simulink library "powerlib_modelsV2"  (Simulink 6.0)
settings: Solver=ode45  SolverMode=SingleTasking  StartTime=0.0  StopTime=10.0  RelTol=1e-3
values from neighbouring files (symbols this model uses):
  Ts = get(handles.edit1,'string')    [powergui.m]
undefined symbols (not defined in the file or in its folder): A, Ac, B, Bc, C, Cc, Cs, Current, damp, Dc, Dd, DiscIntNeverNeededParam, dref, dwo, exc, F, fb, gate, GH, GHd, GI, GId, GL, GLd, H, HT, hyd, ib, ib2, io, isfinite, j, K, Kd, Kg, L, Lad, Laq, lim, LIM, Ll, Llfd, Llkd, Llkq1, Llkq2, Llr, Lls, LowerFlux, N, N2, Nb, Nb2, nb_arm, p, Par_HarmoA_pu, Par_HarmoB_pu, Par_Timing_Harmo, Par_Timing_Variation, Par_Vps, Pb ... (+57)
libraries: powerlib_extras x14
(part 5 of 11)

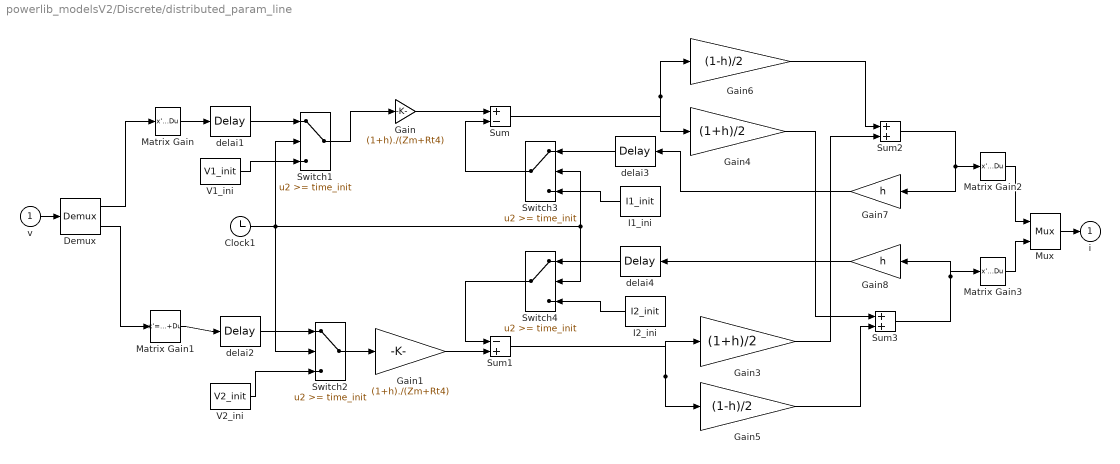
== system powerlib_modelsV2/Discrete/distributed_param_line ==
  v : Inport  Port=1  LatchInput=off
  Clock1 : Clock
      settings: Decimation=10
  Demux : Demux  Outputs=[nphase,nphase]
  Gain : Gain  Gain=(1+h)./(Zm+Rt4)  SaturateOnIntegerOverflow=on
  Gain1 : Gain  Gain=(1+h)./(Zm+Rt4)  SaturateOnIntegerOverflow=on
  Gain3 : Gain  Gain=(1+h)/2  SaturateOnIntegerOverflow=on
  Gain4 : Gain  Gain=(1+h)/2  SaturateOnIntegerOverflow=on
  Gain5 : Gain  Gain=(1-h)/2  SaturateOnIntegerOverflow=on
  Gain6 : Gain  Gain=(1-h)/2  SaturateOnIntegerOverflow=on
  Gain7 : Gain  Orientation=left  Gain=h  SaturateOnIntegerOverflow=on
  Gain8 : Gain  Orientation=left  Gain=h  SaturateOnIntegerOverflow=on
  I1_ini : FromWorkspace  Orientation=left  VariableName=I1_init  SampleTime=0
  I2_ini : FromWorkspace  Orientation=left  VariableName=I2_init  SampleTime=0
  Matrix Gain : StateSpace  A=[]  B=[]  C=[]  D=K  mask(Matrix Gain){@1=Ti'}
      mask prompts: @1 "Gain matrix:"
      mask help: Matrix Gain.
      mask init:
      | K = @1;
      mask Help: Multiplies input vector by entered matrix to produce output vector (y=Au).
      mask Display: disp('K')
  Matrix Gain1 : StateSpace  A=[]  B=[]  C=[]  D=K  mask(Matrix Gain){@1=Ti'}
      mask prompts: @1 "Gain matrix:"
      mask help: Matrix Gain.
      mask init:
      | K = @1;
      mask Help: Multiplies input vector by entered matrix to produce output vector (y=Au).
      mask Display: disp('K')
  Matrix Gain2 : StateSpace  A=[]  B=[]  C=[]  D=K  mask(Matrix Gain){@1=Ti}
      mask prompts: @1 "Gain matrix:"
      mask help: Matrix Gain.
      mask init:
      | K = @1;
      mask Help: Multiplies input vector by entered matrix to produce output vector (y=Au).
      mask Display: disp('K')
  Matrix Gain3 : StateSpace  A=[]  B=[]  C=[]  D=K  mask(Matrix Gain){@1=Ti}
      mask prompts: @1 "Gain matrix:"
      mask help: Matrix Gain.
      mask init:
      | K = @1;
      mask Help: Multiplies input vector by entered matrix to produce output vector (y=Au).
      mask Display: disp('K')
  Mux : Mux  Inputs=[nphase,nphase]
  Sum : Sum  Inputs=+-  SaturateOnIntegerOverflow=on  InputSameDT=on
  Sum1 : Sum  Inputs=-+  SaturateOnIntegerOverflow=on  InputSameDT=on
  Sum2 : Sum  SaturateOnIntegerOverflow=on  InputSameDT=on
  Sum3 : Sum  SaturateOnIntegerOverflow=on  InputSameDT=on
  Switch1 : Switch  Threshold=time_init  InputSameDT=on
  Switch2 : Switch  Threshold=time_init  InputSameDT=on
  Switch3 : Switch  Orientation=left  Threshold=time_init  InputSameDT=on
  Switch4 : Switch  Orientation=left  Threshold=time_init  InputSameDT=on
  V1_ini : FromWorkspace  VariableName=V1_init  SampleTime=0
  V2_ini : FromWorkspace  VariableName=V2_init  SampleTime=0
  delai1 : TransportDelay  DelayTime=to
  delai2 : TransportDelay  DelayTime=to
  delai3 : TransportDelay  Orientation=left  DelayTime=to
  delai4 : TransportDelay  Orientation=left  DelayTime=to
  i : Outport  InitialOutput=0
  wires:
  I2_ini/1 -> Switch4/3
  I1_ini/1 -> Switch3/3
  Clock1/1 -> Switch1/2, Switch2/2, Switch3/2, Switch4/2
  delai4/1 -> Switch4/1
  Switch4/1 -> Sum1/1
  Switch3/1 -> Sum/2
  delai3/1 -> Switch3/1
  Sum1/1 -> Gain5/1, Gain3/1
  Sum/1 -> Gain6/1, Gain4/1
  V2_ini/1 -> Switch2/3
  delai2/1 -> Switch2/1
  Switch1/1 -> Gain/1
  Switch2/1 -> Gain1/1
  V1_ini/1 -> Switch1/3
  delai1/1 -> Switch1/1
  Gain8/1 -> delai4/1
  Sum2/1 -> Matrix Gain2/1, Gain7/1
  Gain7/1 -> delai3/1
  Sum3/1 -> Matrix Gain3/1, Gain8/1
  Mux/1 -> i/1
  v/1 -> Demux/1
  Gain1/1 -> Sum1/2
  Gain/1 -> Sum/1
  Gain5/1 -> Sum3/2
  Gain6/1 -> Sum2/1
  Gain3/1 -> Sum2/2
  Gain4/1 -> Sum3/1
  Matrix Gain/1 -> delai1/1
  Demux/1 -> Matrix Gain/1
  Matrix Gain1/1 -> delai2/1
  Demux/2 -> Matrix Gain1/1
  Matrix Gain3/1 -> Mux/2
  Matrix Gain2/1 -> Mux/1

== system powerlib_modelsV2/Discrete/hysteresis_transformer ==
  v : Inport  Port=1  LatchInput=off
  Hysteresis ( always in SI ) : Subsystem
  fluxinit : DiscreteIntegrator  IntegratorMethod=Integration: Backward Euler  InitialCondition=fluxinit  SampleTime=Ts  SaturateOnIntegerOverflow=on  ICPrevOutput=DiscIntNeverNeededParam  ICPrevScaledInput=DiscIntNeverNeededParam
  i : Outport  InitialOutput=0
  f : Outport  Port=2  InitialOutput=0
  wires:
  v/1 -> fluxinit/1
  fluxinit/1 -> f/1, Hysteresis ( always in SI )/1(In1)  "flux displayed by Multimeter block"
  Hysteresis ( always in SI )/1(Out1) -> i/1

== system powerlib_modelsV2/Discrete/ideal_switch ==
  v : Inport  Port=1  LatchInput=off
  g : Inport  Port=2  LatchInput=off
  0 1 : Constant  Value=0
  Constant : Constant  Value=zeros(Nsw,1)
  Data Type Conversion1 : DataTypeConversion  SaturateOnIntegerOverflow=on  RndMeth=Zero
  Gain : Gain  Gain=1./Rsw  SaturateOnIntegerOverflow=on
  Mux : Mux  Inputs=2
  Switch : Switch  Threshold=0.5  InputSameDT=on
  i : Outport  InitialOutput=0
  Status : Outport  Port=2  InitialOutput=0
  m : Outport  Port=3  InitialOutput=0
  wires:
  v/1 -> Mux/2, Gain/1  "Vak"
  Mux/1 -> m/1  "measurement signals"
  g/1 -> Switch/2, Data Type Conversion1/1
  Constant/1 -> i/1
  Switch/1 -> Mux/1
  Gain/1 -> Switch/1  "Iak"
  0 1/1 -> Switch/3
  Data Type Conversion1/1 -> Status/1

== system powerlib_modelsV2/Discrete/saturable_transformer ==
  v : Inport  Port=1  LatchInput=off
  Discrete-Time Integrator : DiscreteIntegrator  IntegratorMethod=Integration: Trapezoidal  InitialCondition=fluxinit  SampleTime=Ts  SaturateOnIntegerOverflow=on  ICPrevOutput=DiscIntNeverNeededParam  ICPrevScaledInput=DiscIntNeverNeededParam
  Look-Up Table : Lookup  DialogController=Simulink.DDGSource  InputValues=phisat  OutputValues=isat  SaturateOnIntegerOverflow=on
  i : Outport  InitialOutput=0
  f : Outport  Port=2  InitialOutput=0
  wires:
  v/1 -> Discrete-Time Integrator/1
  Discrete-Time Integrator/1 -> Look-Up Table/1, f/1
  Look-Up Table/1 -> i/1

== system powerlib_modelsV2/Discrete/simplified_sync_mach ==
  v : Inport  Port=1  LatchInput=off
  pm : Inport  Port=2  LatchInput=off
  e : Inport  Port=3  LatchInput=off
  1\p : Gain  Gain=1/p  SaturateOnIntegerOverflow=on
  Selector : Selector  Elements=sel  InputPortWidth=3
  Subsystem : Subsystem
  Vt : Subsystem
  Z : Subsystem
      mask Display: disp('Z')
  gen : Subsystem
      mask Display: disp('gen')
  ib : Gain  Gain=ib  SaturateOnIntegerOverflow=on
  mechanics : Subsystem
      mask Display: disp('mec')
  wattmeter : Subsystem  Orientation=left
      mask Display: disp('wattmeter')
  i : Outport  InitialOutput=0
  * : Outport  Port=2  InitialOutput=0
  wires:
  Subsystem/1(*) -> */1
  Vt/2(Vabc) -> Subsystem/2(v), Z/2(v)
  Vt/1(Vn) -> gen/3(Vn)
  gen/1(e) -> wattmeter/2(v), Z/1(e), Subsystem/3(e)  "e"
  Z/1(i) -> wattmeter/1(i), Subsystem/1(i), ib/1
  mechanics/2(wm) -> Subsystem/5(wm)
  1\p/1 -> Subsystem/4(theta)
  v/1 -> Vt/1(V)
  mechanics/1(theta_e) -> gen/1(theta), 1\p/1
  e/1 -> gen/2(E)
  pm/1 -> mechanics/1(Pm)
  wattmeter/1(Pe) -> Subsystem/6(Pe), mechanics/2(Pe)
  ib/1 -> Selector/1
  Selector/1 -> i/1

== system powerlib_modelsV2/Discrete/surge_arrester ==
  v : Inport  Port=1  LatchInput=off
  Abs : Abs  SaturateOnIntegerOverflow=on
  Product : Product  SaturateOnIntegerOverflow=on  InputSameDT=on
  Sign : Signum  Orientation=down
  Switch1 : Switch  Threshold=ic1  InputSameDT=on
  Switch2 : Switch  Threshold=ic2  InputSameDT=on
  Unit Delay1 : UnitDelay  SampleTime=Ts
  segment1 : Fcn  Expr=p1*(u/uref)^a1
  segment2 : Fcn  Expr=p2*(u/uref)^a2
  segment3 : Fcn  Expr=p3*(u/uref)^a3
  i : Outport  InitialOutput=0
  wires:
  segment3/1 -> Switch2/1
  Switch1/1 -> Switch2/3, Switch2/2
  Switch2/1 -> Product/1
  segment2/1 -> Switch1/1
  segment1/1 -> Switch1/2, Switch1/3
  Abs/1 -> segment3/1, segment2/1, segment1/1
  Sign/1 -> Product/2
  v/1 -> Abs/1, Sign/1
  Product/1 -> Unit Delay1/1
  Unit Delay1/1 -> i/1

== system powerlib_modelsV2/Discrete/synchronous_machine ==
  v : Inport  Port=1  LatchInput=off
  pm : Inport  Port=2  LatchInput=off
  vf : Inport  Port=3  LatchInput=off
  Delta angle : Subsystem
  Discrete-Time Integrator1 : DiscreteIntegrator  InitialCondition=tho  SampleTime=Ts  SaturateOnIntegerOverflow=on  ICPrevOutput=DiscIntNeverNeededParam  ICPrevScaledInput=DiscIntNeverNeededParam
  Fcn : Fcn  Expr=rem(u,2*pi)
  Mux1 : Mux  Inputs=[ 3 8 2 4 1 1 1 1 1]
  PQ : Subsystem
  Subsystem : Subsystem
  Unit Delay1 : UnitDelay  Orientation=left  X0=phiqo  SampleTime=Ts
  Unit Delay2 : UnitDelay  Orientation=left  X0=phiqo  SampleTime=Ts
  abc2qd : Subsystem
      mask Display: disp('abc/\nqd')
  currents and mutual fluxes : Subsystem
      mask Display: disp('currents\nand\nmutual\nfluxes')
  ia,ib : Selector  Elements=1:2  InputPortWidth=3
  mec : Subsystem
      mask Display: disp('mec')
  output formatting : Gain  Gain=[ib2*ones(1,5),N2,ib2,ib2,ib2,phib,phib,Vb2,Vb2,1,Nb,Pb,1,1,1,1,1,1]
  phid : Subsystem
      mask Display: disp('phid')
  phifd : Subsystem
      mask Display: disp('phifd')
  phikd : Subsystem
      mask Display: disp('phikd')
  phikq1 : Subsystem
      mask Display: disp('phikq1')
  phikq2 : Subsystem
      mask Display: disp('phikq2')
  phiq : Subsystem
      mask Display: disp('phiq')
  qd2abc : Subsystem
      mask Display: disp('qd/\nabc')
  theta : Gain  Gain=180/pi  SaturateOnIntegerOverflow=on
  vkd : Ground
  vkq2 : Ground
  web1 : Gain  Gain=web_psb  SaturateOnIntegerOverflow=on
  i : Outport  InitialOutput=0
  m : Outport  Port=2  InitialOutput=0
  wires:
  Subsystem/2(Vfd) -> phifd/1(vfd)
  Subsystem/1(Vkq1) -> phikq1/2(vkq1)
  phikq2/1(phikq2) -> currents and mutual fluxes/2(phikq2)
  phikq1/1(phikq1) -> currents and mutual fluxes/5(phikq1)
  phifd/1(phifd) -> currents and mutual fluxes/4(phifd)
  phikd/1(phikd) -> currents and mutual fluxes/6(phikd)
  v/1 -> abc2qd/1(v)
  currents and mutual fluxes/4(phimd) -> Unit Delay2/1
  abc2qd/3(vd) -> phid/3(vd), PQ/2(Vd), Delta angle/2(Vd)
  phid/1(phid) -> mec/2(phid), phiq/3(phid), currents and mutual fluxes/3(phid)
  output formatting/1 -> m/1
  ia,ib/1 -> i/1
  Mux1/1 -> output formatting/1
  currents and mutual fluxes/3(iq,id) -> qd2abc/2(iq,id), mec/1("iq,id "), PQ/3(Iq)  "iq,id"
  abc2qd/1(cos,sin) -> qd2abc/1(sin,cos)  "sin,cos"
  abc2qd/4(vq,vd) -> Mux1/3  "vq,vd"
  qd2abc/2(is(pu)) -> Mux1/1  "is(3)"
  mec/1(misc) -> Mux1/4  "d_theta,n,Pe,dw"
  currents and mutual fluxes/1(phimq) -> Unit Delay1/1
  qd2abc/1(is(A)) -> ia,ib/1  "iabc"
  phiq/1(phiq) -> currents and mutual fluxes/1(phiq), mec/3(phiq), phid/2(phiq)
  vkd/1 -> phikd/2(vkd)
  pm/1 -> mec/4(Pm)
  abc2qd/2(vq) -> phiq/1(vq), PQ/1(Vq), Delta angle/1(Vq)
  vkq2/1 -> phikq2/1(vkq2)
  currents and mutual fluxes/2("iq,id,ifd, ikq1,ikq2,ikd, phimq,phimd") -> Mux1/2  "iq,id,ifd,ikq1,ikq2,ikd,phimq,phimd"
  vf/1 -> Subsystem/1(Vf)
  mec/2(thetae) -> abc2qd/2(theta)
  mec/3(we) -> phid/1(w), phiq/2(w), web1/1
  Fcn/1 -> theta/1
  Discrete-Time Integrator1/1 -> Fcn/1
  web1/1 -> Discrete-Time Integrator1/1
  theta/1 -> Mux1/5  "theta"
  Unit Delay1/1 -> phikq1/1(phimq), phikq2/2(phimq), phiq/4(phimq)
  Unit Delay2/1 -> phifd/2(phimd), phikd/1(phimd), phid/4(phimd)
  mec/4("Te ") -> Mux1/6  "Te"
  Delta angle/1(delta) -> Mux1/7
  PQ/1(Peo) -> Mux1/8
  PQ/2(Qeo) -> Mux1/9

== system powerlib_modelsV2/Discrete/thyristor (logical) ==
  note: Current prediction
  v : Inport  Port=1  LatchInput=off
  g : Inport  Port=2  LatchInput=off
  " Delay Ts1" : UnitDelay  SampleTime=Ts
  " Delay Ts2" : UnitDelay  SampleTime=Ts
  0 {1..4} (4 alike) : Constant  Value=0
  1/Rsw : Gain  Gain=1./Rsw  SaturateOnIntegerOverflow=on
  Constant : Constant  Value=zeros(Nsw,1)
  Data Type  Conversion{1..5} (5 alike) : DataTypeConversion  SaturateOnIntegerOverflow=on  RndMeth=Zero
  Gain : Gain  Gain=2  SaturateOnIntegerOverflow=on
  Mux : Mux  Inputs=2
  Saturation : Saturate  UpperLimit=inf  LowerLimit=0
  Sum : Sum  Inputs=+-  SaturateOnIntegerOverflow=on  InputSameDT=on
  Sum1 : Sum  Inputs=|++  SaturateOnIntegerOverflow=on  InputSameDT=on
  Switch : Switch  Threshold=0.5  InputSameDT=on
  b5 : RelationalOperator  Operator=>  InputSameDT=on
  b6 : RelationalOperator  Operator=>  InputSameDT=on
  b7 : RelationalOperator  Operator===  InputSameDT=on
  or2 : Logic  Operator=OR
  or3 : Logic  Inputs=3
  vf : Constant  Value=Vf
  i : Outport  InitialOutput=0
  Status : Outport  Port=2  InitialOutput=0
  m : Outport  Port=3  InitialOutput=0
  Vf : Outport  Port=4  InitialOutput=0
  wires:
  Mux/1 -> m/1  "measurement signals"
  or3/1 -> or2/2
  Sum/1 -> b5/1
  0 1/1 -> b5/2
  " Delay Ts1"/1 -> Sum/2
  Gain/1 -> Sum/1
  0 2/1 -> b6/2
  v/1 -> b6/1, Sum1/1, 1/Rsw/1  "Vak"
  0 3/1 -> b7/2
  Constant/1 -> i/1
  Sum1/1 -> Mux/2
  vf/1 -> Sum1/2, Vf/1
  or2/1 -> Data Type  Conversion1/1
  Data Type  Conversion1/1 -> " Delay Ts2"/1
  " Delay Ts2"/1 -> Status/1, Switch/2
  g/1 -> Data Type  Conversion2/1
  Data Type  Conversion2/1 -> or3/2
  b6/1 -> Data Type  Conversion3/1
  Data Type  Conversion3/1 -> or3/1
  b7/1 -> Data Type  Conversion4/1
  Data Type  Conversion4/1 -> or3/3
  b5/1 -> Data Type  Conversion5/1
  Data Type  Conversion5/1 -> or2/1
  1/Rsw/1 -> Switch/1  "Iak"
  0 4/1 -> Switch/3
  Switch/1 -> Saturation/1
  Saturation/1 -> Mux/1, b7/1, " Delay Ts1"/1, Gain/1

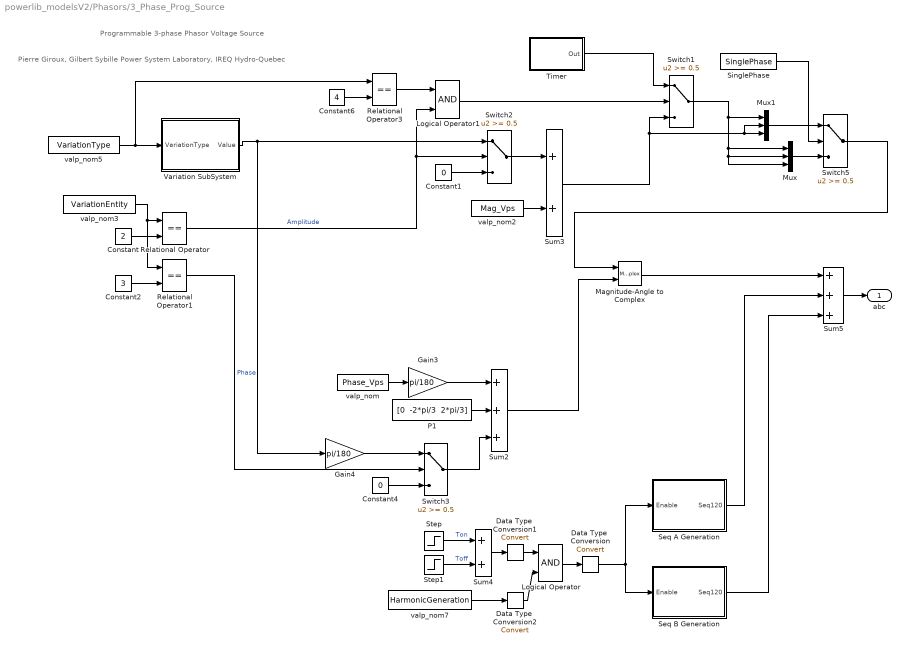
== system powerlib_modelsV2/Phasors/3_Phase_Prog_Source ==
  note: Programmable 3-phase Phasor Voltage Source
  note: Pierre Giroux, Gilbert Sybille
      | Power System Laboratory, IREQ
      | Hydro-Quebec
  Constant : Constant  Value=2
  Constant1 : Constant  Value=0
  Constant2 : Constant  Value=3
  Constant4 : Constant  Value=0
  Constant6 : Constant  Value=4
  Data Type  Conversion : DataTypeConversion  SaturateOnIntegerOverflow=on  RndMeth=Zero
  Data Type  Conversion1 : DataTypeConversion  SaturateOnIntegerOverflow=on  RndMeth=Zero
  Data Type  Conversion2 : DataTypeConversion  SaturateOnIntegerOverflow=on  RndMeth=Zero
  Gain3 : Gain  Gain=pi/180  SaturateOnIntegerOverflow=on
  Gain4 : Gain  Gain=pi/180  SaturateOnIntegerOverflow=on
  Logical Operator : Logic
  Logical Operator1 : Logic
  Magnitude-Angle to Complex : MagnitudeAngleToComplex
  Mux : Mux  Inputs=3
  Mux1 : Mux  Inputs=3
  P1 : Constant  Value="[0  -2*pi/3  2*pi/3]"
  Relational Operator : RelationalOperator  Operator===  InputSameDT=on
  Relational Operator1 : RelationalOperator  Operator===  InputSameDT=on
  Relational Operator3 : RelationalOperator  Operator===  InputSameDT=on
  Seq A Generation : Subsystem  mask(Harmonic generation){Mag_Harmo=Mag_HarmoA *(n_HarmoA==1), Phase_Harmo=Phase_HarmoA, Seq_Harmo=Seq_HarmoA}
  Seq B Generation : Subsystem  mask(Harmonic generation){Mag_Harmo=Mag_HarmoB*(n_HarmoB==1), Phase_Harmo=Phase_HarmoB, Seq_Harmo=Seq_HarmoB}
  SinglePhase : Constant  Value=SinglePhase
  Step : Step  Time=Ton_Harmo  SampleTime=0
  Step1 : Step  Time=Toff_Harmo  After=-1  SampleTime=0
  Sum2 : Sum  Inputs=+++  SaturateOnIntegerOverflow=on  InputSameDT=on
  Sum3 : Sum  SaturateOnIntegerOverflow=on  InputSameDT=on
  Sum4 : Sum  SaturateOnIntegerOverflow=on  InputSameDT=on
  Sum5 : Sum  Inputs=+++  SaturateOnIntegerOverflow=on  InputSameDT=on
  Switch{1..3,5} (4 alike) : Switch  Threshold=0.5  InputSameDT=on
  Timer : Subsystem  mask(Timer){t=Xtime, e=Yampli, Ts=0}
      mask prompts: t "Time (s):"; e "Amplitude:"; Ts "Sample time (s)"
      mask help:
      | Generates a signal changing  at specified times.
      |
      | Value of the signal at time zero must  be specified.
      mask init: same as powerlib_modelsV2/Continuous/3_Phase_Prog_Source/Timer
      mask Display: plot( tv(2:end-1), opv(2:end-1) )
  Variation SubSystem : Subsystem  mask(Variation Subsystem){VariationStep=VariationStep, VariationRate=VariationRate, VariationFreq=VariationFreq, VariationMag=VariationMag, Ton_Variation=Ton_Variation, Toff_Variation=Toff_Variation, Ts=0}
      mask prompts: Ts "Sample time:"
  valp_nom : Constant  Value=Phase_Vps
  valp_nom2 : Constant  Value=Mag_Vps
  valp_nom3 : Constant  Value=VariationEntity
  valp_nom5 : Constant  Value=VariationType
  valp_nom7 : Constant  Value=HarmonicGeneration
  abc : Outport  InitialOutput=0
  wires:
  Data Type  Conversion/1 -> Seq B Generation/1(Enable), Seq A Generation/1(Enable)
  Seq B Generation/1(Seq120) -> Sum5/3
  Seq A Generation/1(Seq120) -> Sum5/2
  Data Type  Conversion2/1 -> Logical Operator/2
  valp_nom7/1 -> Data Type  Conversion2/1
  Data Type  Conversion1/1 -> Logical Operator/1
  Sum4/1 -> Data Type  Conversion1/1
  Logical Operator/1 -> Data Type  Conversion/1
  P1/1 -> Sum2/2
  Magnitude-Angle to Complex/1 -> Sum5/1
  Gain3/1 -> Sum2/1
  valp_nom/1 -> Gain3/1
  Switch2/1 -> Sum3/1
  Constant1/1 -> Switch2/3
  Sum2/1 -> Magnitude-Angle to Complex/2
  valp_nom2/1 -> Sum3/2
  Relational Operator/1 -> Switch2/2, Logical Operator1/2  "Amplitude"
  valp_nom5/1 -> Variation SubSystem/1(VariationType), Relational Operator3/1
  Switch3/1 -> Sum2/3
  Constant4/1 -> Switch3/3
  Relational Operator1/1 -> Switch3/2  "Phase"
  Variation SubSystem/1(Value) -> Gain4/1, Switch2/1
  Constant/1 -> Relational Operator/2
  valp_nom3/1 -> Relational Operator1/1, Relational Operator/1
  Constant2/1 -> Relational Operator1/2
  Step/1 -> Sum4/1  "Ton"
  Step1/1 -> Sum4/2  "Toff"
  Gain4/1 -> Switch3/1
  Constant6/1 -> Relational Operator3/2
  Sum3/1 -> Switch1/3, Mux1/3, Mux1/2
  Timer/1(Out) -> Switch1/1
  Mux1/1 -> Switch5/1
  SinglePhase/1 -> Switch5/2
  Mux/1 -> Switch5/3
  Switch1/1 -> Mux/1, Mux/2, Mux/3, Mux1/1
  Switch5/1 -> Magnitude-Angle to Complex/1
  Relational Operator3/1 -> Logical Operator1/1
  Logical Operator1/1 -> Switch1/2
  Sum5/1 -> abc/1

== system powerlib_modelsV2/Phasors/3_phase_source ==
  Constant : Constant  Value=complex(A*cos(P*pi/180),A*sin(P*pi/180))
  Constant1 : Constant  Value=complex(A*cos((P-120)*pi/180),A*sin((P-120)*pi/180))
  Constant2 : Constant  Value=complex(A*cos((P+120)*pi/180),A*sin((P+120)*pi/180))
  Mux : Mux  Inputs=6
  Sine Wave : Sin  Amplitude=A  Frequency=2*pi*F  Phase=P*pi/180  SampleTime=0
  Sine Wave1 : Sin  Amplitude=A  Frequency=2*pi*F  Phase=(P-120)*pi/180  SampleTime=0
  Sine Wave2 : Sin  Amplitude=A  Frequency=2*pi*F  Phase=(P+120)*pi/180  SampleTime=0
  Out1 : Outport
  wires:
  Mux/1 -> Out1/1
  Constant2/1 -> Mux/6
  Sine Wave2/1 -> Mux/5
  Constant1/1 -> Mux/4
  Sine Wave1/1 -> Mux/3
  Sine Wave/1 -> Mux/1
  Constant/1 -> Mux/2

== system powerlib_modelsV2/Phasors/Dynamic_Load ==
  v : Inport  Port=1  LatchInput=off
  PQ : Inport  Port=2  LatchInput=off
  " filter1" : TransferFcn  Denominator=[1e-3 1]
  Break  Alg. Loop I1 : Subsystem  Orientation=left
  Complex to Real-Imag1 : ComplexToRealImag
  Demux3 : Demux  Outputs=2
  "I1 " : Subsystem
  Mux1 : Mux  Inputs=3
  PQ_ext : Constant  Value=PQext
  Phase currents : Subsystem  Orientation=left
  Power : Subsystem
  Real-Imag to Complex : RealImagToComplex
  Switch1 : Switch  Threshold=0.5  InputSameDT=on
  V> pu : Gain  Gain=1/Vbase  SaturateOnIntegerOverflow=on
  i : Outport  Orientation=left
  m : Outport  Port=2
  wires:
  Phase currents/1(Ia Ib cmplx) -> i/1
  Power/1(P+jQ) -> Switch1/3
  Break  Alg. Loop I1/1(Out) -> Phase currents/1(I1)
  v/1 -> V> pu/1
  "I1 "/1(|V1|) -> " filter1"/1, Power/1(V1)
  V> pu/1 -> "I1 "/1(Vab Vbc cmplx)
  "I1 "/2(I1) -> Break  Alg. Loop I1/1(In)
  " filter1"/1 -> Mux1/1
  Mux1/1 -> m/1
  Complex to Real-Imag1/1 -> Mux1/2
  Complex to Real-Imag1/2 -> Mux1/3
  PQ_ext/1 -> Switch1/2
  Switch1/1 -> "I1 "/2(S=P+jQ), Complex to Real-Imag1/1
  Real-Imag to Complex/1 -> Switch1/1
  Demux3/1 -> Real-Imag to Complex/1
  Demux3/2 -> Real-Imag to Complex/2
  PQ/1 -> Demux3/1

== system powerlib_modelsV2/Phasors/Impedance Measurement ==
  v : Inport  Port=1  LatchInput=off
  Constant : Constant  Value=complex(0,0)
  Terminator : Terminator
  i : Outport  InitialOutput=0
  wires:
  Constant/1 -> i/1
  v/1 -> Terminator/1

== system powerlib_modelsV2/Phasors/asynchronous_machine ==
  note: Note: Model valid only for squirrel cage machine (Vrotor=0)
  note: Ia Ib stator
      | complex
  note: Vab Vbc stator
      | complex
  v : Inport  Port=1  LatchInput=off
  Tm : Inport  Port=2  LatchInput=off
  1_Vb : Gain  Gain=1/Vb  SaturateOnIntegerOverflow=on
  Complex to Magnitude-Angle : ComplexToMagnitudeAngle  Output=Magnitude
  Complex to Magnitude-Angle1 : ComplexToMagnitudeAngle  Output=Magnitude
  Gain : Gain  Gain=[ib2*ones(5,1);phib2;phib2;Vb2;Vb2;ib2*ones(5,1);phib2;phib2;Vb2;Vb2;Nb2;Tb2;1]  SaturateOnIntegerOverflow=on
  Mechanical : Subsystem
  Mux3 : Mux  Inputs=[3,2,2,2,3,2,2,2,3]
  Negative Sequence Model : Subsystem
  Positive Sequence Model : Subsystem
  Selector : Selector  InputPortWidth=3
  Selector1 : Selector  Elements=[1 2]  InputPortWidth=3
  Sum1 : Sum  Inputs=|+-  SaturateOnIntegerOverflow=on  InputSameDT=on
  Sum2 : Sum  Inputs=++|  SaturateOnIntegerOverflow=on  InputSameDT=on
  Vqdr : Constant  Value=[0 0]
  Vqdr1 : Constant  Value=[0 0]
  abc2dq : Subsystem
  dq2abc : Subsystem
  ib : Gain  Gain=ib  SaturateOnIntegerOverflow=on
  ws1 : Constant
  ws2 : Constant
  i : Outport
  m : Outport  Port=2
  wires:
  Negative Sequence Model/2(I2r) -> dq2abc/3(Ir2)
  Negative Sequence Model/1(I2s) -> dq2abc/4(Is2)
  Positive Sequence Model/3(phiqds1) -> Mux3/7  "phiqds1"
  Positive Sequence Model/2(phiqdr1) -> Mux3/3  "phiqdr1"
  abc2dq/2(Vqds2) -> Negative Sequence Model/1(Vqds2)
  Sum2/1 -> Negative Sequence Model/2(s2)  "s2=ws+wr"
  ib/1 -> i/1
  Mux3/1 -> Gain/1
  Gain/1 -> m/1
  dq2abc/2(isabc) -> Complex to Magnitude-Angle1/1, Selector1/1
  dq2abc/1(irabc) -> Complex to Magnitude-Angle/1
  Positive Sequence Model/1(Iqdr1) -> Mux3/2, dq2abc/1(iqdr1)  "iqdr1"
  abc2dq/1(Vqds1) -> Positive Sequence Model/3(Vqds1), Mux3/8  "vqds1"
  Positive Sequence Model/4(Iqds1) -> dq2abc/2(iqds1), Mux3/6  "iqds1"
  Vqdr/1 -> Positive Sequence Model/1(Vqdr1)
  Positive Sequence Model/5(Phiqds1_Isqds1) -> Mechanical/2(phiqds1,iqds1)
  1_Vb/1 -> abc2dq/1(Vab Vbc cmplx)
  v/1 -> 1_Vb/1
  Selector1/1 -> ib/1
  Complex to Magnitude-Angle/1 -> Mux3/1  "irabc"
  Complex to Magnitude-Angle1/1 -> Mux3/5  "isabc"
  Tm/1 -> Mechanical/1(Tm)
  Mechanical/1(wr,Te,thr) -> Selector/1, Mux3/9  "wr, Te, thetam"
  ws1/1 -> Sum1/1
  Sum1/1 -> Positive Sequence Model/2(w-wr)  "s1=ws-wr"
  Vqdr1/1 -> Mux3/4  "Vqdr1"
  ws2/1 -> Sum2/2
  Selector/1 -> Sum2/1, Sum1/2
  Negative Sequence Model/3(Phiqds2_Iqds2) -> Mechanical/3(phiqds2,iqds2)

== system powerlib_modelsV2/Phasors/breaker ==
  "v " : Inport  Port=1  LatchInput=off
  g : Inport  Port=2  LatchInput=off
  Constant : Constant  Value=complex(zeros(Nsw,1),zeros(Nsw,1))
  Terminator : Terminator
  i : Outport  InitialOutput=0
  Status : Outport  Port=2  InitialOutput=0
  wires:
  Constant/1 -> i/1
  g/1 -> Status/1
  "v "/1 -> Terminator/1  "Vak"

== system powerlib_modelsV2/Phasors/distributed_param_line ==
  v : Inport  Port=1  LatchInput=off
  Constant : Constant  Value=complex(zeros(1,2*nphase),zeros(1,2*nphase))
  Terminator : Terminator
  i : Outport  InitialOutput=0
  wires:
  v/1 -> Terminator/1
  Constant/1 -> i/1

== system powerlib_modelsV2/Phasors/ideal_switch ==
  v : Inport  Port=1  LatchInput=off
  g : Inport  Port=2  LatchInput=off
  1/Rsw : Gain  Gain=1./Rsw  SaturateOnIntegerOverflow=on
  1/Rsw1 : Gain  Gain=0  SaturateOnIntegerOverflow=on
  Constant : Constant  Value=complex(zeros(Nsw,1),zeros(Nsw,1))
  Mux : Mux  Inputs=2
  Switch : Switch  Threshold=0.5  InputSameDT=on
  i : Outport  InitialOutput=0
  Status : Outport  Port=2  InitialOutput=0
  m : Outport  Port=3  InitialOutput=0
  wires:
  1/Rsw1/1 -> Switch/3
  Switch/1 -> Mux/1
  1/Rsw/1 -> Switch/1  "Iak"
  v/1 -> Mux/2, 1/Rsw/1, 1/Rsw1/1  "Vak"
  Mux/1 -> m/1  "measurement signals"
  g/1 -> Status/1, Switch/2
  Constant/1 -> i/1

== system powerlib_modelsV2/Phasors/simplified_sync_mach ==
  note: ia ib complex
  note: Vab Vbc
      | complex
  v : Inport  Port=1  LatchInput=off
  pm : Inport  Port=2  LatchInput=off
  e : Inport  Port=3  LatchInput=off
  1_Vb : Gain  Gain=1/Vb  SaturateOnIntegerOverflow=on
  Complex to Magnitude-Angle : ComplexToMagnitudeAngle  Output=Magnitude
  Complex to Magnitude-Angle1 : ComplexToMagnitudeAngle  Output=Magnitude
  Constant4 : Constant  Orientation=left  Value=web
  Filter_T=1ms : StateSpace  A=-1e3*eye(3)  B=1e3*eye(3)  C=eye(3)  D=zeros(3)
  "Idq1 Idq2 Pe " : Subsystem
  Integrator : Integrator  Orientation=left
  LL2LN : Subsystem
  Mux1 : Mux  Inputs=3
  Phasors Ia Ib : Subsystem
  Subsystem : Subsystem
  Sum6 : Sum  Orientation=left  Inputs=+-  SaturateOnIntegerOverflow=on  InputSameDT=on
  ib1 : Gain  Gain=ib  SaturateOnIntegerOverflow=on
  mechanics : Subsystem
      mask Display: disp('mec')
  i : Outport  InitialOutput=0
  m : Outport  Port=2  InitialOutput=0
  wires:
  Mux1/1 -> Subsystem/3(e)
  Complex to Magnitude-Angle1/1 -> Filter_T=1ms/1
  LL2LN/1(Vabc_n) -> Complex to Magnitude-Angle1/1  "Line-to-neutral voltages"
  Complex to Magnitude-Angle/1 -> Subsystem/1(i)
  Phasors Ia Ib/1(Iabc cmplx) -> Complex to Magnitude-Angle/1
  mechanics/1(theta_e) -> Sum6/1  "delta"
  "Idq1 Idq2 Pe "/1(Pe) -> Subsystem/6(Pe), mechanics/2(Pe)  "Pe"
  Sum6/1 -> Subsystem/4(theta), "Idq1 Idq2 Pe "/3(delta)  "theta"
  mechanics/2(wm) -> Subsystem/5(wm)  "w"
  Integrator/1 -> Sum6/2
  Constant4/1 -> Integrator/1
  ib1/1 -> i/1
  Phasors Ia Ib/2(Iab cmplx) -> ib1/1
  e/1 -> Mux1/3, Mux1/1, Mux1/2, "Idq1 Idq2 Pe "/2(e)  "Internal volltage  magnitudes"
  1_Vb/1 -> LL2LN/1(Vab_bc), "Idq1 Idq2 Pe "/1(Vab Vbc cmplx)
  v/1 -> 1_Vb/1
  Subsystem/1(*) -> m/1
  pm/1 -> mechanics/1(Pm)
  "Idq1 Idq2 Pe "/2(Idq1) -> Phasors Ia Ib/1(Idq1)
  "Idq1 Idq2 Pe "/3(Idq2) -> Phasors Ia Ib/2(Idq2)
  Filter_T=1ms/1 -> Subsystem/2(v)

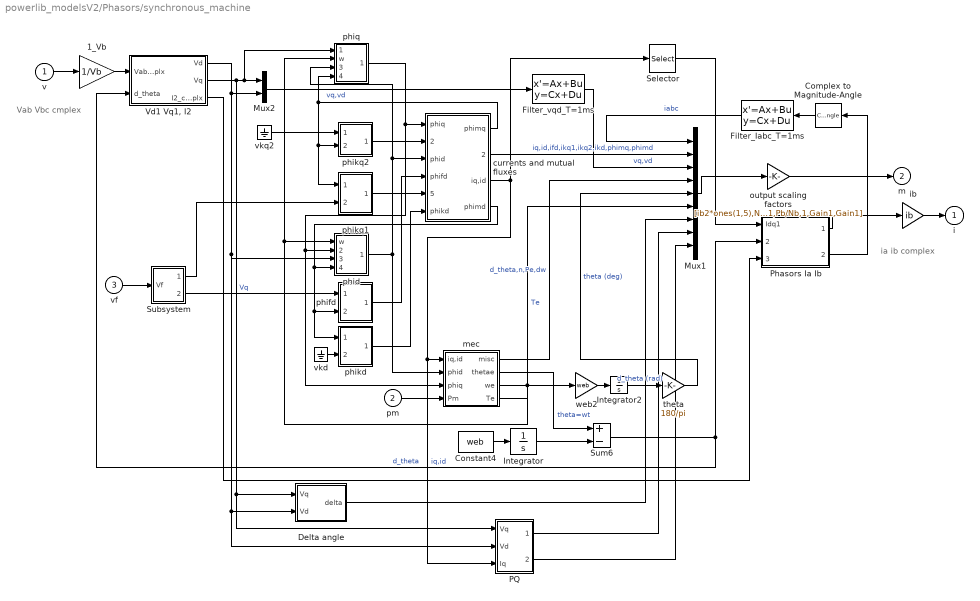
== system powerlib_modelsV2/Phasors/synchronous_machine ==
  note: Vab Vbc cmplex
  note: ia ib complex
  v : Inport  Port=1  LatchInput=off
  pm : Inport  Port=2  LatchInput=off
  vf : Inport  Port=3  LatchInput=off
  1_Vb : Gain  Gain=1/Vb  SaturateOnIntegerOverflow=on
  Complex to Magnitude-Angle : ComplexToMagnitudeAngle  Orientation=left  Output=Magnitude
  Constant4 : Constant  Value=web
  Delta angle : Subsystem
  Filter_Iabc_T=1ms : StateSpace  Orientation=left  A=-1e3*eye(3)  B=1e3*eye(3)  C=eye(3)  D=zeros(3)
  Filter_vqd_T=1ms : StateSpace  A=-1e3*eye(2)  B=1e3*eye(2)  C=eye(2)  D=zeros(2)  X0=[phido -phiqo]
  Integrator : Integrator
  Integrator2 : Integrator  InitialCondition=tho
  Mux1 : Mux  Inputs=[ 3 8 2 4 1 1 1 1 1]
  Mux2 : Mux  Inputs=2
  PQ : Subsystem
  Phasors Ia Ib : Subsystem
  Selector : Selector  Elements=[2 1]  InputPortWidth=2
  Subsystem : Subsystem
  Sum6 : Sum  Inputs=+-  SaturateOnIntegerOverflow=on  InputSameDT=on
  "Vd1 Vq1, I2 " : Subsystem
  currents and mutual fluxes : Subsystem
  ib : Gain  Gain=ib  SaturateOnIntegerOverflow=on
  mec : Subsystem
  output scaling factors : Gain  Gain=[ib2*ones(1,5),N2,ib2,ib2,ib2,phib,phib,Vb2,Vb2,1,Nb,Pb,1,1,Pb/Nb,1,Gain1,Gain1]
  phid : Subsystem
      mask Display: disp('phid')
  phifd : Subsystem
      mask Display: disp('phifd')
  phikd : Subsystem
      mask Display: disp('phikd')
  phikq1 : Subsystem
      mask Display: disp('phikq1')
  phikq2 : Subsystem
      mask Display: disp('phikq2')
  phiq : Subsystem
      mask Display: disp('phiq')
  theta : Gain  Gain=180/pi  SaturateOnIntegerOverflow=on
  vkd : Ground
  vkq2 : Ground
  web2 : Gain  Gain=web  SaturateOnIntegerOverflow=on
  i : Outport  InitialOutput=0
  m : Outport  Port=2  InitialOutput=0
  wires:
  PQ/2(Qeo) -> Mux1/9
  PQ/1(Peo) -> Mux1/8
  Delta angle/1(delta) -> Mux1/7
  theta/1 -> Mux1/5  "theta (deg)"
  Integrator2/1 -> theta/1  "d_theta (rad)"
  web2/1 -> Integrator2/1
  Complex to Magnitude-Angle/1 -> Filter_Iabc_T=1ms/1
  Phasors Ia Ib/2(Iabc cmplx) -> Complex to Magnitude-Angle/1
  ib/1 -> i/1
  Phasors Ia Ib/1(Ia Ib cmplx) -> ib/1
  mec/3(we) -> web2/1, phiq/2(w), phid/1(w)
  currents and mutual fluxes/1(phimq) -> phiq/4(phimq), phikq1/1(phimq), phikq2/2(phimq)
  currents and mutual fluxes/4(phimd) -> phid/4(phimd), phifd/2(phimd), phikd/1(phimd)
  phiq/1(phiq) -> mec/3(phiq), phid/2(phiq), currents and mutual fluxes/1(phiq)
  "Vd1 Vq1, I2 "/1(Vd) -> Delta angle/2(Vd), PQ/2(Vd), phid/3(vd), Mux2/2
  "Vd1 Vq1, I2 "/2(Vq) -> Delta angle/1(Vq), PQ/1(Vq), phiq/1(vq), Mux2/1  "Vq"
  phid/1(phid) -> phiq/3(phid), currents and mutual fluxes/3(phid), mec/2(phid)
  Selector/1 -> Phasors Ia Ib/1(Idq1)
  Mux2/1 -> Filter_vqd_T=1ms/1  "vq,vd"
  "Vd1 Vq1, I2 "/3(I2_cmplx) -> Phasors Ia Ib/3(I2_cmplx)
  mec/2(thetae) -> Sum6/1  "theta=wt"
  Integrator/1 -> Sum6/2
  Constant4/1 -> Integrator/1
  Sum6/1 -> Phasors Ia Ib/2(d_theta), "Vd1 Vq1, I2 "/2(d_theta)  "d_theta"
  phikq2/1(phikq2) -> currents and mutual fluxes/2(phikq2)
  phikq1/1(phikq1) -> currents and mutual fluxes/5(phikq1)
  phifd/1(phifd) -> currents and mutual fluxes/4(phifd)
  phikd/1(phikd) -> currents and mutual fluxes/6(phikd)
  output scaling factors/1 -> m/1
  Mux1/1 -> output scaling factors/1
  currents and mutual fluxes/3(iq,id) -> mec/1("iq,id "), PQ/3(Iq), Selector/1  "iq,id"
  mec/1(misc) -> Mux1/4  "d_theta,n,Pe,dw"
  pm/1 -> mec/4(Pm)
  currents and mutual fluxes/2("iq,id,ifd, ikq1,ikq2,ikd, phimq,phimd") -> Mux1/2  "iq,id,ifd,ikq1,ikq2,ikd,phimq,phimd"
  v/1 -> 1_Vb/1
  1_Vb/1 -> "Vd1 Vq1, I2 "/1(Vab Vbc cmplx)
  Subsystem/2(Vfd) -> phifd/1(vfd)
  Subsystem/1(Vkq1) -> phikq1/2(vkq1)
  vkd/1 -> phikd/2(vkd)
  vkq2/1 -> phikq2/1(vkq2)
  vf/1 -> Subsystem/1(Vf)
  mec/4("Te ") -> Mux1/6  "Te"
  Filter_Iabc_T=1ms/1 -> Mux1/1  "iabc"
  Filter_vqd_T=1ms/1 -> Mux1/3  "vq,vd"

== system powerlib_modelsV2/Switch Current Source/IGBT ==
  v : Inport  Port=1  LatchInput=off
  g : Inport  Port=2  LatchInput=off
  Conduction Logic : Subsystem
  IC : InitialCondition  Value=IC
  Integrator : Integrator  ExternalReset=rising  InitialConditionSource=external  ShowStatePort=on
  L_device : Gain  Gain=1./Lon  SaturateOnIntegerOverflow=on
  Mux : Mux  Inputs=2
  R_device : Gain  Orientation=left  Gain=Ron  SaturateOnIntegerOverflow=on
  Switch : Switch  Threshold=eps  InputSameDT=on
  Tail : Subsystem
  Vak-VT-RT*Iak2 : Sum  Inputs=-|+|-  SaturateOnIntegerOverflow=on  InputSameDT=on
  Vf : Constant  Orientation=up  Value=Vf
  Vf1 : Constant  Value=0*IC
  Vf2 : Constant  Value=0
  i : Outport  InitialOutput=0
  m : Outport  Port=2  InitialOutput=0
  wires:
  Conduction Logic/1(status) -> Tail/2(switch), Integrator/2, Switch/2
  Integrator/1 -> R_device/1, Tail/1(iak)  "IGBT current"
  IC/1 -> Integrator/3
  Integrator/State -> Conduction Logic/1(iak)  "IGBT current"
  g/1 -> Conduction Logic/3(g)  "gate signal"
  Vak-VT-RT*Iak2/1 -> L_device/1
  Tail/1(Iak) -> Mux/1, i/1  "current"
  Mux/1 -> m/1
  Vf/1 -> Vak-VT-RT*Iak2/3
  v/1 -> Vak-VT-RT*Iak2/2, Conduction Logic/2(Vak), Mux/2  "IGBT voltage"
  R_device/1 -> Vak-VT-RT*Iak2/1
  Vf1/1 -> IC/1
  Switch/1 -> Integrator/1
  L_device/1 -> Switch/1
  Vf2/1 -> Switch/3

== system powerlib_modelsV2/Switch Current Source/detailed_thyristor ==
  v : Inport  Port=1  LatchInput=off
  g : Inport  Port=2  LatchInput=off
  Conduction logic : Subsystem
  Mux : Mux  Inputs=2
  Switch-Ron-Lon : Subsystem
  i : Outport  InitialOutput=0
  m : Outport  Port=2  InitialOutput=0
  wires:
  Conduction logic/1(reset) -> Switch-Ron-Lon/2(Reset)
  Mux/1 -> m/1
  Switch-Ron-Lon/1("Iak  ") -> i/1, Mux/1, Conduction logic/1(Iak_meas.)
  v/1 -> Switch-Ron-Lon/1(Vak), Conduction logic/2(Vak), Mux/2
  g/1 -> Conduction logic/3(G)

== system powerlib_modelsV2/Switch Current Source/diode ==
  v : Inport  Port=1  LatchInput=off
  0  1 : Constant  Value=0
  Conduction logic : Subsystem
  IC : InitialCondition  Value=IC
  Integrator1 : Integrator  ExternalReset=rising  InitialConditionSource=external  LimitOutput=on  LowerSaturationLimit=0
  Lon : Gain  Gain=1./Lon  SaturateOnIntegerOverflow=on
  Mux : Mux  Inputs=2
  Ron : Gain  Orientation=left  Gain=Ron  SaturateOnIntegerOverflow=on
  Test : Switch  Threshold=0.5  InputSameDT=on
  Vak-VT-RT*Iak2 : Sum  Inputs=-|+|-  SaturateOnIntegerOverflow=on  InputSameDT=on
  Vf : Constant  Orientation=up  Value=Vf
  Vf1 : Constant  Value=0*IC
  i : Outport  InitialOutput=0
  m : Outport  Port=2  InitialOutput=0
  wires:
  Mux/1 -> m/1
  v/1 -> Mux/2, Conduction logic/2(Vak), Vak-VT-RT*Iak2/2  "Diode voltage"
  IC/1 -> Integrator1/3
  Lon/1 -> Integrator1/1
  Conduction logic/1(status) -> Integrator1/2, Test/2
  Vak-VT-RT*Iak2/1 -> Lon/1
  Integrator1/1 -> Ron/1, Test/1  "Inductor current"
  Ron/1 -> Vak-VT-RT*Iak2/1
  Vf/1 -> Vak-VT-RT*Iak2/3
  Vf1/1 -> IC/1
  0  1/1 -> Test/3  "zero current"
  Test/1 -> i/1, Mux/1, Conduction logic/1(Iak)  "Diode current"

== system powerlib_modelsV2/Switch Current Source/gto ==
  v : Inport  Port=1  LatchInput=off
  g : Inport  Port=2  LatchInput=off
  Conduction Logic : Subsystem
  IC : InitialCondition  Value=IC
  Integrator : Integrator  ExternalReset=rising  InitialConditionSource=external  ShowStatePort=on
  L_device : Gain  Gain=1./Lon  SaturateOnIntegerOverflow=on
  Mux : Mux  Inputs=2
  R_device : Gain  Orientation=left  Gain=Ron  SaturateOnIntegerOverflow=on
  Switch : Switch  Threshold=eps  InputSameDT=on
  Tail : Subsystem
  Vak-VT-RT*Iak2 : Sum  Inputs=-|+|-  SaturateOnIntegerOverflow=on  InputSameDT=on
  Vf : Constant  Orientation=up  Value=Vf
  Vf1 : Constant  Value=0*IC
  Vf2 : Constant  Value=0
  i : Outport  InitialOutput=0
  m : Outport  Port=2  InitialOutput=0
  wires:
  Conduction Logic/1(status) -> Tail/2(switch), Integrator/2, Switch/2  "switch status"
  Integrator/1 -> Tail/1(iak), R_device/1  "GTO current"
  Integrator/State -> Conduction Logic/1(iak)  "GTO current"
  g/1 -> Conduction Logic/3(g)  "gate signal"
  R_device/1 -> Vak-VT-RT*Iak2/1
  Tail/1(Iak) -> i/1, Mux/1  "GTO current"
  Mux/1 -> m/1
  v/1 -> Vak-VT-RT*Iak2/2, Mux/2, Conduction Logic/2(Vak)  "GTO voltage"
  Vf/1 -> Vak-VT-RT*Iak2/3
  Vak-VT-RT*Iak2/1 -> L_device/1
  Vf1/1 -> IC/1
  IC/1 -> Integrator/3
  Switch/1 -> Integrator/1
  L_device/1 -> Switch/1
  Vf2/1 -> Switch/3

== system powerlib_modelsV2/Switch Current Source/mosfet ==
  v : Inport  Port=1  LatchInput=off
  g : Inport  Port=2  LatchInput=off
  0  1 : Constant  Value=0
  Conduction Logic : Subsystem
  IC : InitialCondition  Value=IC
  Integrator1 : Integrator  ExternalReset=rising  InitialConditionSource=external  LowerSaturationLimit=0  ShowStatePort=on
  Lon : Gain  Gain=1./Lon  SaturateOnIntegerOverflow=on
  Mux : Mux  Inputs=2
  R_device : Gain  Orientation=left  Gain=Ron  SaturateOnIntegerOverflow=on
  R_device1 : Gain  Orientation=left  Gain=Rd  SaturateOnIntegerOverflow=on
  Sign : Signum  Orientation=left
  Test : Switch  Threshold=0.5  InputSameDT=on
  Test4 : Switch  Orientation=left  Threshold=eps  InputSameDT=on
  Vds-Ron*Ids : Sum  Inputs=-+|  SaturateOnIntegerOverflow=on  InputSameDT=on
  Vf1 : Constant  Value=0*IC
  i : Outport  InitialOutput=0
  m : Outport  Port=2  InitialOutput=0
  wires:
  Integrator1/1 -> Test/1, Sign/1, R_device/1, R_device1/1  "mosfet current"
  Test/1 -> Mux/1, i/1
  Conduction Logic/1(status) -> Integrator1/2, Test/2
  Integrator1/State -> Conduction Logic/1(Ids_meas)  "mosfet current"
  v/1 -> Mux/2, Conduction Logic/2(Vds), Vds-Ron*Ids/2  "mosfet voltage"
  Sign/1 -> Test4/2
  R_device1/1 -> Test4/3
  Lon/1 -> Integrator1/1
  Vds-Ron*Ids/1 -> Lon/1
  R_device/1 -> Test4/1
  g/1 -> Conduction Logic/3(G)  "gate signal"
  Mux/1 -> m/1
  Test4/1 -> Vds-Ron*Ids/1
  0  1/1 -> Test/3  "zero current"
  Vf1/1 -> IC/1
  IC/1 -> Integrator1/3

== system powerlib_modelsV2/Switch Current Source/thyristor ==
  v : Inport  Port=1  LatchInput=off
  g : Inport  Port=2  LatchInput=off
  0  1 : Constant  Value=0
  Conduction Logic : Subsystem
  IC : InitialCondition  Value=IC
  Integrator : Integrator  ExternalReset=rising  InitialConditionSource=external  LimitOutput=on  LowerSaturationLimit=0
  Lon : Gain  Gain=1./Lon  SaturateOnIntegerOverflow=on
  Mux : Mux  Inputs=2
  R_device : Gain  Orientation=left  Gain=Ron  SaturateOnIntegerOverflow=on
  Test : Switch  Threshold=0.5  InputSameDT=on
  Vak-VT-RT*Iak2 : Sum  Inputs=-|+|-  SaturateOnIntegerOverflow=on  InputSameDT=on
  Vf : Constant  Orientation=up  Value=Vf
  Vf1 : Constant  Value=0*IC
  i : Outport  InitialOutput=0
  m : Outport  Port=2  InitialOutput=0
  wires:
  g/1 -> Conduction Logic/3("G ")  "gate signal"
  Conduction Logic/1(Status) -> Integrator/2, Test/2
  Mux/1 -> m/1
  Lon/1 -> Integrator/1
  Integrator/1 -> R_device/1, Test/1  "Inductor current"
  v/1 -> Conduction Logic/2(Vak), Mux/2, Vak-VT-RT*Iak2/2  "thyristor voltage"
  Vak-VT-RT*Iak2/1 -> Lon/1
  IC/1 -> Integrator/3
  R_device/1 -> Vak-VT-RT*Iak2/1
  Vf/1 -> Vak-VT-RT*Iak2/3
  Vf1/1 -> IC/1
  Test/1 -> i/1, Mux/1, Conduction Logic/1("Iak ")  "Thyiristor Current"
  0  1/1 -> Test/3  "zero current"

== system powerlib_modelsV2/Continuous/3_Phase_Prog_Source/Harmonic A generation ==
  Enable : Inport  Port=1  LatchInput=off
  Clock : Clock
  Gain2 : Gain  Gain=2*pi*n_Harmo  SaturateOnIntegerOverflow=on
  Gain3 : Gain  Gain=pi/180  SaturateOnIntegerOverflow=on
  Multiport Switch : MultiPortSwitch  Inputs=3  InputSameDT=on
  Negative-sequence : Constant  Value=[0 2*pi/3 -2*pi/3]
  Phase_Harmo : Constant  Value=Phase_Harmo
  Phase_Harmo1 : Constant  Value=Mag_Harmo
  Phase_Harmo2 : Constant  Value=Seq_Harmo
  Positive-sequence : Constant  Value=[0 -2*pi/3 2*pi/3]
  Product : Product  SaturateOnIntegerOverflow=on  InputSameDT=on
  Product1 : Product  Inputs=3  SaturateOnIntegerOverflow=on  InputSameDT=on
  Sum : Sum  Inputs=+++  SaturateOnIntegerOverflow=on  InputSameDT=on
  Sum1 : Sum  SaturateOnIntegerOverflow=on  InputSameDT=on
  Trigonometric Function1 : Trigonometry
  Zero-sequence : Constant  Value=[0 0 0]
  valp_nom1 : Constant  Value=Freq_Vps
  valp_nom2 : Constant
  HarmoA : Outport
  wires:
  Gain3/1 -> Sum/2
  Phase_Harmo/1 -> Gain3/1
  Enable/1 -> Product1/1
  valp_nom2/1 -> Sum1/2
  Phase_Harmo2/1 -> Sum1/1
  Sum1/1 -> Multiport Switch/1
  Phase_Harmo1/1 -> Product1/2
  Product1/1 -> HarmoA/1
  Trigonometric Function1/1 -> Product1/3
  Product/1 -> Sum/1
  Clock/1 -> Product/1
  Gain2/1 -> Product/2
  valp_nom1/1 -> Gain2/1
  Negative-sequence/1 -> Multiport Switch/4
  Positive-sequence/1 -> Multiport Switch/3
  Zero-sequence/1 -> Multiport Switch/2
  Multiport Switch/1 -> Sum/3
  Sum/1 -> Trigonometric Function1/1

== system powerlib_modelsV2/Continuous/3_Phase_Prog_Source/Harmonic B generation ==
  Enable : Inport  Port=1  LatchInput=off
  Clock1 : Clock
  Gain2 : Gain  Gain=2*pi*n_Harmo  SaturateOnIntegerOverflow=on
  Gain3 : Gain  Gain=pi/180  SaturateOnIntegerOverflow=on
  Multiport Switch : MultiPortSwitch  Inputs=3  InputSameDT=on
  Negative-sequence : Constant  Value=[0 2*pi/3 -2*pi/3]
  Phase_Harmo : Constant  Value=Phase_Harmo
  Phase_Harmo1 : Constant  Value=Mag_Harmo
  Phase_Harmo2 : Constant  Value=Seq_Harmo
  Positive-sequence : Constant  Value=[0 -2*pi/3 2*pi/3]
  Product : Product  SaturateOnIntegerOverflow=on  InputSameDT=on
  Product1 : Product  Inputs=3  SaturateOnIntegerOverflow=on  InputSameDT=on
  Sum : Sum  Inputs=+++  SaturateOnIntegerOverflow=on  InputSameDT=on
  Sum1 : Sum  SaturateOnIntegerOverflow=on  InputSameDT=on
  Trigonometric Function1 : Trigonometry
  Zero-sequence : Constant  Value=[0 0 0]
  valp_nom1 : Constant  Value=Freq_Vps
  valp_nom2 : Constant
  HarmoB : Outport
  wires:
  Gain3/1 -> Sum/2
  Phase_Harmo/1 -> Gain3/1
  Sum/1 -> Trigonometric Function1/1
  Multiport Switch/1 -> Sum/3
  Zero-sequence/1 -> Multiport Switch/2
  Positive-sequence/1 -> Multiport Switch/3
  Negative-sequence/1 -> Multiport Switch/4
  valp_nom1/1 -> Gain2/1
  Gain2/1 -> Product/2
  Clock1/1 -> Product/1
  Product/1 -> Sum/1
  Trigonometric Function1/1 -> Product1/3
  Product1/1 -> HarmoB/1
  Phase_Harmo1/1 -> Product1/2
  Sum1/1 -> Multiport Switch/1
  Phase_Harmo2/1 -> Sum1/1
  valp_nom2/1 -> Sum1/2
  Enable/1 -> Product1/1

== system powerlib_modelsV2/Continuous/3_Phase_Prog_Source/Timer ==
  Clock : Clock
  Look-Up Table : Lookup  DialogController=Simulink.DDGSource  InputValues=tv  OutputValues=opv  SaturateOnIntegerOverflow=on
  Out : Outport
  wires:
  Look-Up Table/1 -> Out/1
  Clock/1 -> Look-Up Table/1

== system powerlib_modelsV2/Continuous/3_Phase_Prog_Source/Variation SubSystem ==
  VariationType : Inport  Port=1  LatchInput=off
  Constant : Constant  Value=2
  Constant1 : Constant  Value=0
  Constant2 : Constant
  Constant3 : Constant
  Constant4 : Constant  Value=0
  Constant5 : Constant  Value=0
  Data Type  Conversion1 : DataTypeConversion  SaturateOnIntegerOverflow=on  RndMeth=Zero
  Data Type  Conversion2 : DataTypeConversion  Orientation=up  SaturateOnIntegerOverflow=on  RndMeth=Zero
  Gain1 : Gain  Gain=2*pi  SaturateOnIntegerOverflow=on
  Integrator : Integrator
  Logical Operator : Logic
  Logical Operator1 : Logic  Orientation=up  Operator=NOT
  Memory : Memory  Orientation=left
  Multiport Switch1 : MultiPortSwitch  InputSameDT=on
  Product : Product  SaturateOnIntegerOverflow=on  InputSameDT=on
  Product1 : Product  SaturateOnIntegerOverflow=on  InputSameDT=on
  Product2 : Product  SaturateOnIntegerOverflow=on  InputSameDT=on
  Relational Operator : RelationalOperator  Operator===  InputSameDT=on
  Relational Operator1 : RelationalOperator  Operator===  InputSameDT=on
  Step : Step  Time=Ton_Variation  SampleTime=0
  Step1 : Step  Time=Toff_Variation  Before=1  After=0  SampleTime=0
  Switch{,1..3} (4 alike) : Switch  Threshold=0.5  InputSameDT=on
  Trigonometric Function1 : Trigonometry
  valp_nom6 : Constant  Value=VariationStep
  valp_nom7 : Constant  Value=VariationRate
  valp_nom8 : Constant  Value=VariationMag
  valp_nom9 : Constant  Value=VariationFreq
  Value : Outport
  wires:
  Data Type  Conversion1/1 -> Logical Operator/2
  Constant5/1 -> Multiport Switch1/5
  Logical Operator1/1 -> Logical Operator/1
  Logical Operator/1 -> Switch3/2
  Step1/1 -> Switch2/2, Data Type  Conversion2/1  "Toff"
  Constant3/1 -> Relational Operator1/2
  Switch3/1 -> Value/1
  Switch2/1 -> Switch3/3, Memory/1
  Constant1/1 -> Switch3/1
  Memory/1 -> Switch2/3
  Multiport Switch1/1 -> Switch2/1
  Step/1 -> Product2/2, Switch/2  "Ton"
  VariationType/1 -> Relational Operator/1, Relational Operator1/1, Multiport Switch1/1
  Integrator/1 -> Multiport Switch1/3, Product1/1  "Ramp"
  Product2/1 -> Multiport Switch1/2  "Step"
  valp_nom6/1 -> Product2/1
  Relational Operator/1 -> Switch1/2
  Switch/1 -> Integrator/1
  Constant/1 -> Relational Operator/2
  Switch1/1 -> Switch/1
  Constant4/1 -> Switch/3
  Constant2/1 -> Switch1/3
  valp_nom7/1 -> Switch1/1
  Product/1 -> Multiport Switch1/4  "Mod"
  Product1/1 -> Trigonometric Function1/1
  Gain1/1 -> Product1/2
  valp_nom9/1 -> Gain1/1
  valp_nom8/1 -> Product/1
  Trigonometric Function1/1 -> Product/2
  Data Type  Conversion2/1 -> Logical Operator1/1
  Relational Operator1/1 -> Data Type  Conversion1/1

== system powerlib_modelsV2/Continuous/Dynamic_Load/3-phase PLL1 ==
  note: 3-phase PLL
  note: Pierre Giroux, Gilbert Sybille
      | Power System Laboratory, IREQ
      | Hydro-Quebec
  Vab_bc (pu) : Inport  Port=1  PortDimensions=2  LatchInput=off
  2nd-Order Filter : Subsystem  AncestorBlock=|  mask(2nd-Order Filter){FilterType=Lowpass, Fo=25, Zeta=0.707, Initialize=on, Vac_Init=[0 0 60], Vdc_Init=Finit, PlotResponse=off, param1=[1 1000 0.5]}
      | powerlib_extras/Control 
      | Blocks/2nd-Order
      | Filter
      mask prompts: FilterType "Filter Type:"; Fo "Cut-off frequency (Hz):"; Zeta "Damping factor Zeta ( Q = 1 / (2*Zeta) ):"; Initialize "Initialize filter states"; Vac_Init "AC initial input: [ Mag  Phase(degrees)  Freq(Hz) ]"; Vdc_Init "DC Initial input:"; PlotResponse "Plot filter response"; param1 "Frequency range(Hz) : [Start  End  Inc.]"
      mask init:
      | Wo=2*pi*Fo;
      | str=sprintf(' Fo=%iHz\n\n',Fo);
      | switch FilterType
      | case 1, % Lowpass
      |        X=[0 1 2 3 4];
      |        Y=[-2 -2 -3 -4 -4];
      |        n2=0;n1=0;n0=Wo*Wo;
      |        d2=1;d1=2*Zeta*Wo;d0=Wo*Wo;
      |  case 2,   % Highpass
      |        X=[0 1 2 3 4];
      |        Y=[-4 -4 -3 -2 -2];
      |        n2=1;n1=0;n0=0;
      |        d2=1;d1=2*Zeta*Wo;d0=Wo*Wo;
      |     case 3,   % Bandpass
      |        X=[0 1 2 3 4 5 ];
      |        Y=[-3 -3 -2 -2 -3 -3];
      |        n2=0;n1=2*Zeta*Wo;n0=0;
      |        d2=1;d1=2*Zeta*Wo;d0=Wo*Wo;
      |     case 4,  %Bandstop (Notch)
      |        X=[0 1 2 3 4 5 ];
      |        Y=[-2 -2 -3 -3 -2 -2];
      |        n2=1;n1=0;n0=Wo*Wo;
      |        d2=1;d1=2*Zeta*Wo;d0=Wo*Wo;
      |     end
      | %
      | numc=[n2 n1 n0];
      | denc=[d2 d1 d0];
      | [Ac,Bc,Cc,Dc]=tf2ss(numc,denc);
      | %
      | if Initialize==1  % Compute initial conditions on states
      | u1=Vac_Init(1)*exp(j*Vac_Init(2)*pi/180);
      | u2=Vdc_Init*exp(j*90*pi/180);
      | u=u1+u2;
      | u0=imag(u); % input at  t=0;
      | I=eye(size(Ac));
      | sI1=I*j*(2*pi*Vac_Init(3));
      | sI2=I*j*0;
      | x=inv(sI1-Ac)*Bc*u1 + inv(sI2-Ac)*Bc*u2;
      | x0c=imag(x);
      | else
      | x0c=0;
      | end
      | %
      | if PlotResponse==1 % Plot frequency and step response
      | figure(1)
      | sys=ss(Ac,Bc,Cc,Dc);
      | f=param1(1):param1(3):param1(2);
      | w=2*pi*f;
      | [mag phase]=bode(sys,w);
      | subplot(2,1,1)
      | plot(f,squeeze(mag))
      | title('Magnitude')
      | grid
      | subplot(2,1,2)
      | plot(f,squeeze(phase))
      | title('Phase (degrees)')
      | xlabel('Hz')
      | grid
      | figure(2)
      | step(sys)
      | end
      mask StyleString: popup(Lowpass|Highpass|Bandpass|Bandstop (Notch)),edit,edit,checkbox,edit,edit,checkbox,edit
      mask CallbackString: |||parametres=get_param(gcb,'MaskValues');p4=parametres{4};p7=parametres{7};if strcmp(p4,'on');param5='on';param6='on';else;param5='off';param6='off';end;if strcmp(p7,'on');param8='on';else;param8='off';end;visible={'on','on','on','on',param5,param6,'on',param8};set_param(gcb,'MaskVisibilities',visible)|||parametres=get_param(gcb,'MaskValues');p4=parametres{4};p7=parametres{7};if strcmp(p4,'on');param5='on';param6='on';else;param5='off';param6='off';end;if strcmp(p7,'on');param8='on';else;param8='off';end;visible={'on','on','on','on',param5,param6,'on',param8};set_param(gcb,'MaskVisibilities',visible)|
      mask Display:
      | plot(X,Y);
      | disp(str);
  Constant4 : Constant  Value=2*pi
  Discrete PI Controller : Subsystem  mask(Discrete PI Controller){Kp=Kp, Ki=Ki, Par_Limits=2*pi*Finit*[1.25 0.75], Init=2*pi*Finit}
      mask prompts: Kp "Proportional gain (Kp):"; Ki "Integral gain (Ki):"; Par_Limits "Output limits: [ Upper   Lower ]"; Init "Output initial value:"
      mask help: This block implements a discrete PI controller.
      mask init:
      | UpperLimit=Par_Limits(1);
      | LowerLimit=Par_Limits(2);
      mask Display: disp('PI');
  Gain10 : Gain  Gain=1/2/pi  SaturateOnIntegerOverflow=on
  Integrator : Integrator  InitialCondition=Phase_Init*pi/180  LimitOutput=on
  Math Function : Math  Operator=mod  SaturateOnIntegerOverflow=on
  Mux2 : Mux  Inputs=2
  Rate Limiter : RateLimiter  RisingSlewLimit=12  FallingSlewLimit=-12
  Trigonometric Function : Trigonometry
  Trigonometric Function2 : Trigonometry  Operator=cos
  Variable Frequency Mean value : Subsystem  mask(Variable-Frequency Mean Value){Finit=Finit, Vinit=0}
      mask prompts: Finit "Initial frequency (Hz):"; Vinit "Initial input (DC component):"
      mask help:
      | This  block computes the mean value of the input signal (port In) over a running window of one cycle of a specified frequency (port Freq).
      |
      | For the first cycle of simulation (specified by the parameter "Initial frequency"), the ouput is held to the value of the  "Initial input" parameter.
  abc_to_dq1 : Subsystem
  Freq : Outport
  Vd : Outport  Port=2
  Vq : Outport  Port=3
  Sin_Cos : Outport  Port=4
  wires:
  abc_to_dq1/1(vd) -> Vd/1
  2nd-Order Filter/1(Out) -> Freq/1, Variable Frequency Mean value/1(Freq)
  Variable Frequency Mean value/1(Mean) -> Discrete PI Controller/1(Error)
  Vab_bc (pu)/1 -> abc_to_dq1/1(Vab_bc)
  abc_to_dq1/2(vq) -> Vq/1, Variable Frequency Mean value/2(In)  "Vq"
  Constant4/1 -> Math Function/2
  Integrator/1 -> Math Function/1
  Math Function/1 -> Trigonometric Function/1, Trigonometric Function2/1
  Trigonometric Function/1 -> Mux2/1
  Trigonometric Function2/1 -> Mux2/2
  Mux2/1 -> abc_to_dq1/2(sin_cos), Sin_Cos/1
  Discrete PI Controller/1(Out) -> Integrator/1, Gain10/1  "W"
  Gain10/1 -> Rate Limiter/1
  Rate Limiter/1 -> 2nd-Order Filter/1(In)
